simulink subsystem "modelo_LTI_equivalente_aumentado"  (R2023b)
settings: Solver=VariableStepAuto  StartTime=0.0  StopTime=10.0  RelTol=1e-3
values from neighbouring files (symbols this model uses):
  b_eq = 2.1944e-5    (= 2.1944e-05)    [diagrama_polos_y_ceros_LTI.m]    (also in main.m = 2.19444444444e-05; parametros.m = 2.19444444444e-05)
  C_ts = 0.818    [parametros.m]
  J_eq = 1.9785e-5    (= 1.9785e-05)    [diagrama_polos_y_ceros_LTI.m]    (also in main.m = 1.97847222222e-05; parametros.m = 1.97847222222e-05)
  L_d = 6.6    [main.m]    (also in parametros.m = 0.0066)
  L_Is = 0.8    [main.m]    (also in parametros.m = 0.0008)
  L_q = 5.8e-3    (= 0.0058)    [diagrama_polos_y_ceros_LTI.m]    (also in main.m = 5.8; parametros.m; variacion_de_parametros.m)
  lambda_m = 0.016    [main.m]    (also in parametros.m)
  P_p = 3    [diagrama_polos_y_ceros_LTI.m]    (also in main.m; parametros.m; variacion_de_parametros.m)
  r = 120.0    (= 120)    [diagrama_polos_y_ceros_LTI.m]    (also in main.m; parametros.m)
  R_s = R_sref    (= 1.02)    [parametros.m]
  R_sref = 1.02    [parametros.m]
  R_tsamb = 146.7    [parametros.m]
settings Model: Creator=nicol  LastModifiedBy=Julya

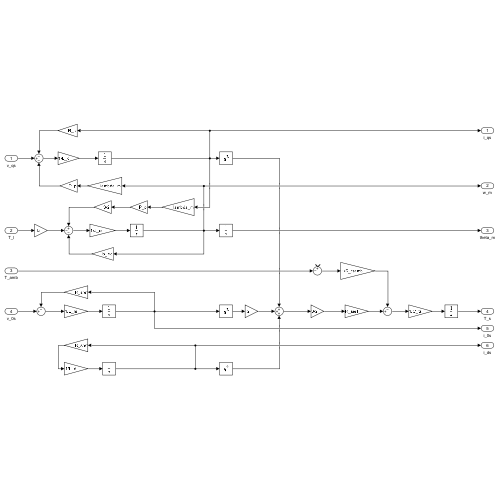
[thumbnail: Simulink's stored preview of the top-level diagram]
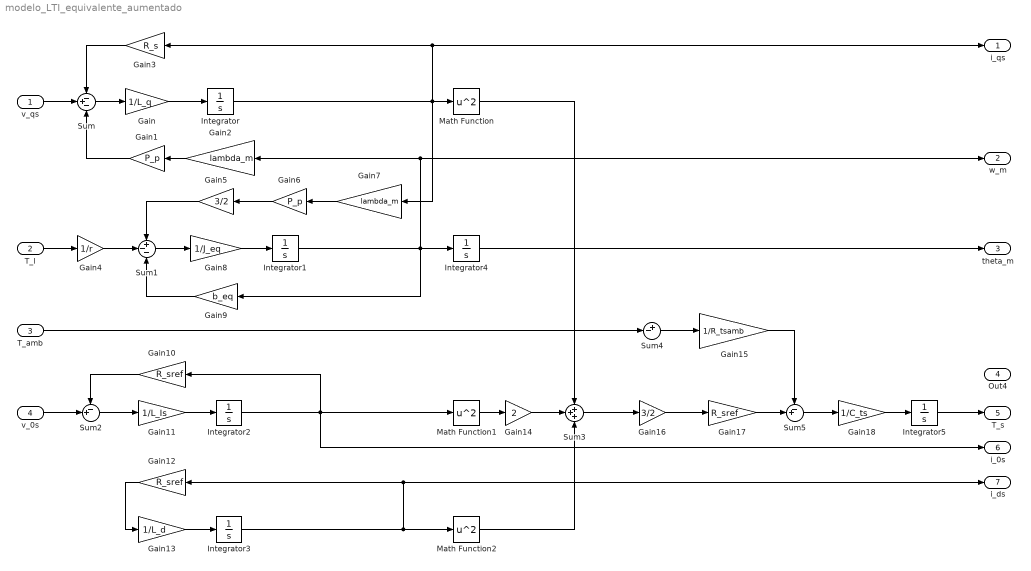
== system modelo_LTI_equivalente_aumentado ==
  v_qs : Inport
  T_l : Inport  Port=2
  T_amb : Inport  Port=3
  v_0s : Inport  Port=4
  Gain : Gain  Gain=1/L_q
  Gain1 : Gain  Gain=P_p
  Gain10 : Gain  Gain=R_sref
  Gain11 : Gain  Gain=1/L_Is
  Gain12 : Gain  Gain=R_sref
  Gain13 : Gain  Gain=1/L_d
  Gain14 : Gain  Gain=2
  Gain15 : Gain  Gain=1/R_tsamb
  Gain16 : Gain  Gain=3/2
  Gain17 : Gain  Gain=R_sref
  Gain18 : Gain  Gain=1/C_ts
  Gain2 : Gain  Gain=lambda_m
  Gain3 : Gain  Gain=R_s
  Gain4 : Gain  Gain=1/r
  Gain5 : Gain  Gain=3/2
  Gain6 : Gain  Gain=P_p
  Gain7 : Gain  Gain=lambda_m
  Gain8 : Gain  Gain=1/J_eq
  Gain9 : Gain  Gain=b_eq
  Integrator{,1..5} (6 alike) : Integrator
  Math Function : Math  Operator=square
  Math Function1 : Math  Operator=square
  Math Function2 : Math  Operator=square
  Sum : Sum  Inputs=-+-
  Sum1 : Sum  Inputs=+--
  Sum2 : Sum  Inputs=-+|
  Sum3 : Sum  Inputs=+++
  Sum4 : Sum  Inputs=+-|
  Sum5 : Sum  Inputs=-+|
  i_qs : Outport
  w_m : Outport  Port=2
  theta_m : Outport  Port=3
  Out4 : Outport  Port=4
  T_s : Outport  Port=5
  i_0s : Outport  Port=6
  i_ds : Outport  Port=7
  wires:
  Gain1/1 -> Sum/3
  Gain3/1 -> Sum/1
  Sum/1 -> Gain/1
  Gain/1 -> Integrator/1
  Gain2/1 -> Gain1/1
  v_qs/1 -> Sum/2
  Sum1/1 -> Gain8/1
  Gain8/1 -> Integrator1/1
  Gain9/1 -> Sum1/3
  Gain5/1 -> Sum1/1
  Gain6/1 -> Gain5/1
  Gain7/1 -> Gain6/1
  Gain4/1 -> Sum1/2
  T_l/1 -> Gain4/1
  v_0s/1 -> Sum2/2
  Gain10/1 -> Sum2/1
  Sum2/1 -> Gain11/1
  Gain11/1 -> Integrator2/1
  Gain13/1 -> Integrator3/1
  Gain12/1 -> Gain13/1
  Integrator/1 -> Gain7/1, i_qs/1, Gain3/1, Math Function/1
  Integrator1/1 -> w_m/1, Gain2/1, Gain9/1, Integrator4/1
  Integrator2/1 -> Gain10/1, i_0s/1, Math Function1/1
  Integrator3/1 -> i_ds/1, Gain12/1, Math Function2/1
  Math Function1/1 -> Gain14/1
  Math Function2/1 -> Sum3/3
  Gain14/1 -> Sum3/2
  Math Function/1 -> Sum3/1
  T_amb/1 -> Sum4/2
  Gain17/1 -> Sum5/2
  Sum4/1 -> Gain15/1
  Gain15/1 -> Sum5/1
  Sum5/1 -> Gain18/1
  Gain18/1 -> Integrator5/1
  Gain16/1 -> Gain17/1
  Sum3/1 -> Gain16/1
  Integrator5/1 -> T_s/1
  Integrator4/1 -> theta_m/1
